simulink model "sim5"  (R2022b)
settings: Solver=VariableStepAuto  StartTime=0.0  StopTime=czas_symulacji  RelTol=1e-3
values from neighbouring files (symbols this model uses):
  dqg = 0.1*qgN    (= 1000)    [lab5.m]
  dTzew = 0    [lab5.m]
  L_11 = [Cvp, Kcwp + Kcp]    [lab5.m]
  L_12 = [Cvp*Kcw, Kcwp*Kcw + Kcp*Kcw + Kcwp]    [lab5.m]
  L_21 = Kcwp    (= 69.7674418605)    [lab5.m]
  L_22 = [Cv*Kcp, Kcw*Kcwp + Kcw*Kcp + Kcwp*Kcp]    [lab5.m]
  M = [Cvp*Cv, Cvp*Kcw+Cvp*Kcwp+Cv*Kcwp+Cv*Kcp, Kcwp*Kcw + Kcp*Kcw + Kcp*Kcwp]    [lab5.m]
  t0 = 500    [lab5.m]
  Tp0 = (Tzew0*(Kcwp*Kcp+Kcwp*Kcw+Kcw*Kcp)+Kcwp*qg0)/(Kcwp*Kcp+Kcwp*Kcw+Kcw*Kcp)    (= 10)    [lab5.m]
  Twew0 = (qg0+(Tzew0*Kcw)+(Tp0*Kcwp))/(Kcwp+Kcw)    (= 20)    [lab5.m]
settings Model: Creator=Gosia  LastModifiedBy=Gosia
settings DataIOCC: ReturnWorkspaceOutputs=off

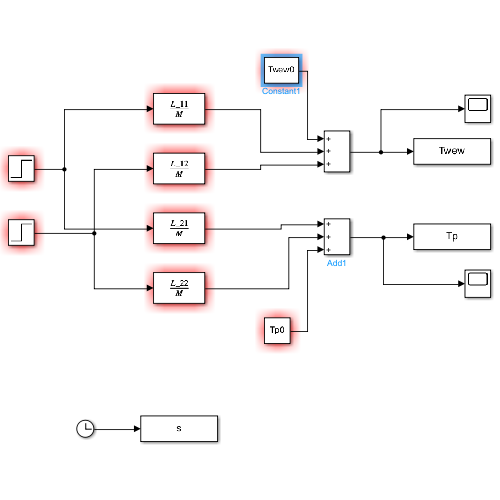
[thumbnail: Simulink's stored preview of the top-level diagram]
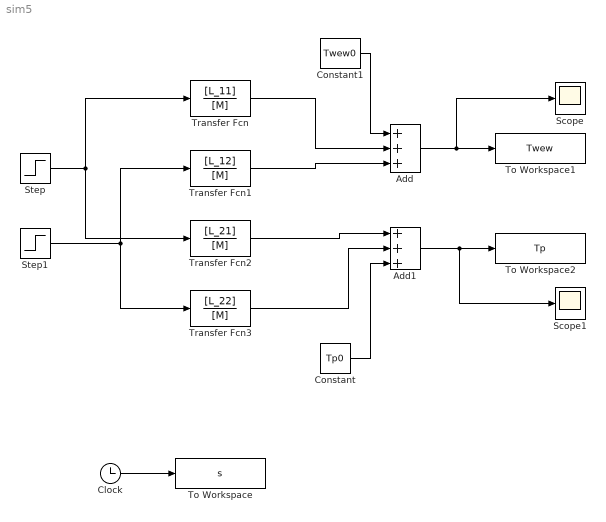
== system sim5 ==
  Add : Sum  Inputs=+++
  Add1 : Sum  Inputs=+++
  Clock : Clock
  Constant : Constant  Value=Tp0
  Constant1 : Constant  Value=Twew0
  Scope : Scope
  Scope1 : Scope
  Step : Step  Time=t0  After=dqg  SampleTime=0
  Step1 : Step  Time=t0  After=dTzew  SampleTime=0
  To Workspace : ToWorkspace  VariableName=s  SaveFormat=Timeseries  SampleTime=-1
  To Workspace1 : ToWorkspace  VariableName=Twew  SampleTime=-1
  To Workspace2 : ToWorkspace  VariableName=Tp  SampleTime=-1
  Transfer Fcn : TransferFcn  Numerator=[L_11]  Denominator=[M]
  Transfer Fcn1 : TransferFcn  Numerator=[L_12]  Denominator=[M]
  Transfer Fcn2 : TransferFcn  Numerator=[L_21]  Denominator=[M]
  Transfer Fcn3 : TransferFcn  Numerator=[L_22]  Denominator=[M]
  wires:
  Clock/1 -> To Workspace/1
  Transfer Fcn2/1 -> Add1/1
  Add/1 -> Scope/1, To Workspace1/1
  Transfer Fcn3/1 -> Add1/2
  Add1/1 -> Scope1/1, To Workspace2/1
  Step1/1 -> Transfer Fcn1/1, Transfer Fcn3/1
  Step/1 -> Transfer Fcn2/1, Transfer Fcn/1
  Transfer Fcn1/1 -> Add/3
  Transfer Fcn/1 -> Add/2
  Constant/1 -> Add1/3
  Constant1/1 -> Add/1
